simulink model "GCI_Ctrl_PLL_C2000"  (R2024a)
settings: Solver=FixedStepDiscrete  StartTime=0.0  StopTime=8  FixedStep=Sim.ContSampleTime  RelTol=1e-3  EnableMultiTasking=on
values from neighbouring files (symbols this model uses):
  ADPTV = 1.3912    [ModelDD.sldd]
  Ctrl = 0    [ModelDD.sldd]
  EnableMonitors = 0    [ModelDD.sldd]
  FrcPwr = 1    [ModelDD.sldd]
  IdSp = 0.0    [ModelDD.sldd]
  IqSp = 0.0    [ModelDD.sldd]
  ModReq = 1    [ModelDD.sldd]
  PorISel = 0    [ModelDD.sldd]
  PSp = 0.0    [ModelDD.sldd]
  QSp = 0.0    [ModelDD.sldd]
  Sim : value not decoded    [ModelDD.sldd]
  Test = 0    [ModelDD.sldd]
  Var = 650.0    [ModelDD.sldd]
undefined symbols (not defined in the file or in its folder): DiscIntNeverNeededParam, Down, GPTRIP1SEL, GPTRIP2SEL, magnitude, P, TZ1, TZ2, Up
libraries: simulink x38, c2837xDlib x22, c2802xlib x15, slpidlib x9, spsMeanLib x9, spsCurrentMeasurementLib x7, spsThreePhaseVIMeasurementLib x5, spsVoltageMeasurementLib x5, spsTHDLib x4, spsSeriesRLCBranchLib x4, svdutilitieslib x3, c280xlib x3
(part 8 of 11)

== system GCI_Ctrl_PLL_C2000/C2000_SW/CtrlLoop/CurrentController/CurrentControllerAdptv2/MESO/Mag1 ==
  in : Inport
  Gain : Gain  Gain=4
  Gain1 : Gain  Gain=0.5
  Product : Product
  Product1 : Product
  Selector : Selector  NumberOfDimensions=2  InputPortWidth=3  IndexOptions=Index vector (dialog),Index vector (dialog)  Indices=1,1  OutputSizes=1,1
  Selector1 : Selector  NumberOfDimensions=2  InputPortWidth=3  IndexOptions=Index vector (dialog),Index vector (dialog)  Indices=2,2  OutputSizes=1,1
  Selector2 : Selector  NumberOfDimensions=2  InputPortWidth=3  IndexOptions=Index vector (dialog),Index vector (dialog)  Indices=1,2  OutputSizes=1,1
  Selector3 : Selector  NumberOfDimensions=2  InputPortWidth=3  IndexOptions=Index vector (dialog),Index vector (dialog)  Indices=2,1  OutputSizes=1,1
  Sqrt1 : Sqrt
  Sqrt2 : Sqrt
  Square : Math  Operator=square
  Square1 : Math  Operator=square
  Square2 : Math  Operator=square
  Sum : Sum  Inputs=|+-
  Sum of Elements : Sum  Inputs=+
  Sum1 : Sum  Inputs=|+-
  Sum2 : Sum  Inputs=|+-
  Abs : Outport
  wires:
  Sqrt2/1 -> Abs/1
  Gain1/1 -> Sqrt2/1
  Sum2/1 -> Gain1/1
  Sqrt1/1 -> Sum2/2
  Sum1/1 -> Sqrt1/1
  Gain/1 -> Sum1/2
  Square1/1 -> Sum1/1
  Square2/1 -> Gain/1
  [det] -> Square2/1
  Sum/1 -> [det]
  Product1/1 -> Sum/2
  Product/1 -> Sum/1
  Selector2/1 -> Product1/1
  Selector3/1 -> Product1/2
  Selector1/1 -> Product/2
  Selector/1 -> Product/1
  Sum of Elements/1 -> Square1/1, Sum2/1
  in/1 -> Square/1, Selector/1, Selector3/1, Selector2/1, Selector1/1
  Square/1 -> Sum of Elements/1

== system GCI_Ctrl_PLL_C2000/C2000_SW/CtrlLoop/CurrentController/CurrentControllerAdptv2/MESO/Mag2 ==
  in : Inport
  Constant : Constant  OutDataTypeStr=single
  Fcn : Fcn  Expr=(u[2]+sqrt(u[2]^2 - 4*u[1]*u[3]))/(2*u[1])
  Fcn1 : Fcn  Expr=(u[2]-sqrt(u[2]^2 - 4*u[1]*u[3]))/(2*u[1])
  Matrix Multiply : Product  Multiplication=Matrix(*)
  Max : MinMax  Function=max  Inputs=2
  Mux : Mux  Inputs=3
  Product : Product
  Product1 : Product
  Reshape{,1..4} (5 alike) : Reshape
  Selector : Selector  NumberOfDimensions=2  InputPortWidth=3  IndexOptions=Index vector (dialog),Index vector (dialog)  Indices=1,1  OutputSizes=1,1
  Selector1 : Selector  NumberOfDimensions=2  InputPortWidth=3  IndexOptions=Index vector (dialog),Index vector (dialog)  Indices=1,2  OutputSizes=1,1
  Selector2 : Selector  NumberOfDimensions=2  InputPortWidth=3  IndexOptions=Index vector (dialog),Index vector (dialog)  Indices=2,1  OutputSizes=1,1
  Selector3 : Selector  NumberOfDimensions=2  InputPortWidth=3  IndexOptions=Index vector (dialog),Index vector (dialog)  Indices=2,2  OutputSizes=1,1
  Sqrt3 : Sqrt
  Sum : Sum  Inputs=|++
  Sum1 : Sum  Inputs=|+-
  Transpose : matrix_library/Transpose
  Abs : Outport
  wires:
  Matrix Multiply/1 -> Selector/1, Selector1/1, Selector2/1, Selector3/1
  Constant/1 -> Mux/1
  Sum1/1 -> Mux/3
  Product1/1 -> Sum1/2
  Product/1 -> Sum1/1
  Sum/1 -> Mux/2
  Fcn1/1 -> Max/2
  Fcn/1 -> Max/1
  Mux/1 -> Fcn/1, Fcn1/1
  Reshape4/1 -> Sum/2, Product1/2  "d"
  Reshape3/1 -> Product/2  "c"
  Reshape2/1 -> Product/1  "b"
  Selector1/1 -> Reshape2/1
  Selector2/1 -> Reshape3/1
  Selector3/1 -> Reshape4/1
  Reshape1/1 -> Sum/1, Product1/1  "a"
  Selector/1 -> Reshape1/1
  Sqrt3/1 -> Reshape/1
  Max/1 -> Sqrt3/1
  in/1 -> Transpose/1, Matrix Multiply/2
  Transpose/1 -> Matrix Multiply/1
  Reshape/1 -> Abs/1

== system GCI_Ctrl_PLL_C2000/C2000_SW/CtrlLoop/CurrentController/CurrentControllerAdptv2/MESO/Subsystem ==
  $v_k$ : Inport
  "$u_{k-1}$" : Inport  Port=2
  Abs : Abs  SaturateOnIntegerOverflow=off
  Constant : Constant  Value=ADPTV.b_D_ui
  Constant1 : Constant  Value=ADPTV.b_D_ui
  Less Than : RelationalOperator  Operator=<  OutDataTypeStr=boolean  RndMeth=Simplest  InputSameDT=off
  Product : Product
  Sign : Signum
  Sum6 : Sum  Inputs=|++
  Switch : Switch  Criteria=u2 > Threshold  SaturateOnIntegerOverflow=off  InputSameDT=off
  $u_k$ : Outport
  wires:
  "$u_{k-1}$"/1 -> Sum6/2
  Sum6/1 -> $u_k$/1  "$u_k$"
  Switch/1 -> Sum6/1
  Abs/1 -> Less Than/1
  Constant1/1 -> Product/2
  Product/1 -> Switch/3
  Constant/1 -> Less Than/2
  $v_k$/1 -> Switch/1, Abs/1, Sign/1
  Less Than/1 -> [ui_cond]  "$u_{sat}$"
  [ui_cond] -> Switch/2
  Sign/1 -> Product/1

== system GCI_Ctrl_PLL_C2000/C2000_SW/CtrlLoop/CurrentController/CurrentControllerAdptv2/Subsystem/PowerCalculation ==
  VdqP : Inport
  VdqN : Inport  Port=2
  IdqzP : Inport  Port=3
  IdqzN : Inport  Port=4
  Add : Sum  Inputs=-+
  Add3 : Sum
  Add4 : Sum
  Demux : Demux  Outputs=2
  Gain4 : Gain  Gain=1.5  ParamDataTypeStr=single
  Gain5 : Gain  Gain=1.5  ParamDataTypeStr=single
  Product{4..7} (4 alike) : Product
  Selector2 : Selector  InputPortWidth=2  IndexOptions=Index vector (dialog)  Indices=[2 1]  OutputSizes=1
  Selector3 : Selector  InputPortWidth=2  IndexOptions=Index vector (dialog)  Indices=[2 1]  OutputSizes=1
  Sum of Elements3 : Sum  Inputs=+
  P0 : Outport  VectorParamsAs1DForOutWhenUnconnected=off
  Q0 : Outport  Port=2  VectorParamsAs1DForOutWhenUnconnected=off
  wires:
  IdqzP/1 -> [IdqP], Selector2/1
  VdqN/1 -> [VdqN]
  IdqzN/1 -> [IdqN], Selector3/1
  VdqP/1 -> [VdqP]
  Product5/1 -> Add3/2
  Add3/1 -> Demux/1
  Product4/1 -> Add3/1
  Add/1 -> Gain4/1
  Gain4/1 -> Q0/1
  Selector2/1 -> [IqdP]
  Selector3/1 -> [IqdN]
  [IqdP] -> Product4/2
  [VdqP] -> Product4/1
  [IqdN] -> Product5/2
  [VdqN] -> Product5/1
  [VdqN] -> Product7/1
  [IdqN] -> Product7/2
  [VdqP] -> Product6/1
  [IdqP] -> Product6/2
  Gain5/1 -> P0/1
  Sum of Elements3/1 -> Gain5/1
  Product6/1 -> Add4/1
  Add4/1 -> Sum of Elements3/1
  Product7/1 -> Add4/2
  Demux/1 -> Add/1
  Demux/2 -> Add/2

== system GCI_Ctrl_PLL_C2000/C2000_SW/CtrlLoop/CurrentController/CurrentControllerAdptv2/Subsystem/abc_dqz ==
  abc : Inport
  wtNow : Inport  Port=2
  Subsystem : Subsystem
  Subsystem2 : Subsystem
  dqz : Outport  VectorParamsAs1DForOutWhenUnconnected=off
  wires:
  wtNow/1 -> Subsystem2/2(Ang)
  abc/1 -> Subsystem/1(abc)
  Subsystem/1(al_be_0) -> Subsystem2/1(alpha_beta)
  Subsystem2/1(dq) -> dqz/1

== system GCI_Ctrl_PLL_C2000/C2000_SW/CtrlLoop/CurrentController/CurrentControllerAdptv2/Subsystem/abc_dqz1 ==
  abc : Inport
  wtNow : Inport  Port=2
  Subsystem : Subsystem
  Subsystem2 : Subsystem
  dqz : Outport  VectorParamsAs1DForOutWhenUnconnected=off
  wires:
  Subsystem2/1(dq) -> dqz/1
  Subsystem/1(al_be_0) -> Subsystem2/1(alpha_beta)
  abc/1 -> Subsystem/1(abc)
  wtNow/1 -> Subsystem2/2(Ang)

== system GCI_Ctrl_PLL_C2000/C2000_SW/CtrlLoop/CurrentController/CurrentControllerAdptv2/Subsystem/dd_dqz1 ==
  abc : Inport
  wtNow : Inport  Port=2
  Delay : Delay  DelayLength=1
  Delay1 : Delay  DelayLength=1
  Gain : Gain  Gain=-1  ParamDataTypeStr=single
  LPF : Subsystem  mask{Ts=1/(Var.PWM_Freq), w=single(2*pi*50), K=single(1), y_0=0}
      mask prompts: Ts "Sample Time (s)"; w "CutOff Freq (-3db) (rad/s)"; K "Gain"; y_0 "Initial output"
  LPF1 : Subsystem  mask{Ts=1/(Var.PWM_Freq), w=single(2*pi*50), K=single(1), y_0=0}
      mask prompts: Ts "Sample Time (s)"; w "CutOff Freq (-3db) (rad/s)"; K "Gain"; y_0 "Initial output"
  Subsystem : Subsystem
  Subsystem1 : Subsystem
  Subsystem2 : Subsystem
  Subsystem3 : Subsystem
  Subsystem4 : Subsystem
  dqzP : Outport  VectorParamsAs1DForOutWhenUnconnected=off
  dqzN : Outport  Port=2  VectorParamsAs1DForOutWhenUnconnected=off
  wires:
  Subsystem1/1(dq) -> Subsystem3/1(Vdq_in)
  Subsystem2/1(dq) -> Subsystem4/1(Vdq_in)
  Subsystem4/1(Vdq_out) -> LPF/1(u), dqzP/1
  Delay/1 -> Subsystem3/2(Vdq_Inverse)
  Delay1/1 -> Subsystem4/2(Vdq_Inverse)
  Subsystem3/1(Vdq_out) -> LPF1/1(u), dqzN/1
  LPF1/1(y) -> Delay1/1
  LPF/1(y) -> Delay/1
  Gain/1 -> Subsystem1/2(wtNow), Subsystem3/3(Theta)
  abc/1 -> Subsystem/1(abc)
  Subsystem/1(al_be_0) -> Subsystem2/1(alpha_beta), Subsystem1/1(alpha_beta)
  wtNow/1 -> Gain/1, Subsystem2/2(wtNow), Subsystem4/3(Theta)

== system GCI_Ctrl_PLL_C2000/C2000_SW/CtrlLoop/CurrentController/CurrentControllerAdptv2/Subsystem/dd_dqz2 ==
  abc : Inport
  wtNow : Inport  Port=2
  Delay : Delay  DelayLength=1
  Delay1 : Delay  DelayLength=1
  Gain : Gain  Gain=-1  ParamDataTypeStr=single
  LPF : Subsystem  mask{Ts=1/(Var.PWM_Freq), w=single(50), K=single(1), y_0=0}
      mask prompts: Ts "Sample Time (s)"; w "CutOff Freq (-3db) (rad/s)"; K "Gain"; y_0 "Initial output"
  LPF1 : Subsystem  mask{Ts=1/(Var.PWM_Freq), w=single(50), K=single(1), y_0=0}
      mask prompts: Ts "Sample Time (s)"; w "CutOff Freq (-3db) (rad/s)"; K "Gain"; y_0 "Initial output"
  Subsystem : Subsystem
  Subsystem1 : Subsystem
  Subsystem2 : Subsystem
  Subsystem3 : Subsystem
  Subsystem4 : Subsystem
  dqzP : Outport  VectorParamsAs1DForOutWhenUnconnected=off
  dqzN : Outport  Port=2  VectorParamsAs1DForOutWhenUnconnected=off
  wires:
  Subsystem/1(al_be_0) -> Subsystem1/1(alpha_beta), Subsystem2/1(alpha_beta)
  abc/1 -> Subsystem/1(abc)
  Gain/1 -> Subsystem3/3(Theta), Subsystem1/2(wtNow)
  LPF/1(y) -> Delay/1
  LPF1/1(y) -> Delay1/1
  Subsystem3/1(Vdq_out) -> LPF1/1(u), dqzN/1
  Delay1/1 -> Subsystem4/2(Vdq_Inverse)
  Delay/1 -> Subsystem3/2(Vdq_Inverse)
  Subsystem4/1(Vdq_out) -> LPF/1(u), dqzP/1
  Subsystem2/1(dq) -> Subsystem4/1(Vdq_in)
  Subsystem1/1(dq) -> Subsystem3/1(Vdq_in)
  wtNow/1 -> Gain/1, Subsystem4/3(Theta), Subsystem2/2(wtNow)

== system GCI_Ctrl_PLL_C2000/C2000_SW/CtrlLoop/CurrentController/CurrentControllerAdptv2/dqz2abc_1/Subsystem ==
  al_be_0 : Inport  OutDataTypeStr=single  PortDimensions=3
  Gain3 : Gain  Gain="single([ 1   0   1; -1/2  sqrt(3)/2   1; -1/2  -sqrt(3)/2  1 ] )"  Multiplication=Matrix(K*u) (u vector)  ParamDataTypeStr=single  OutDataTypeStr=single  SaturateOnIntegerOverflow=on
  abc : Outport  OutDataTypeStr=single  VectorParamsAs1DForOutWhenUnconnected=off
  wires:
  al_be_0/1 -> Gain3/1
  Gain3/1 -> abc/1  "abc"

== system GCI_Ctrl_PLL_C2000/C2000_SW/CtrlLoop/CurrentController/CurrentControllerAdptv2/dqz2abc_1/Subsystem1 ==
  note: =
  note: =
  note: *
  note: [ d
      |    q ]
  note: [  al
      |     be  ]
  note: [ d
      |    q ]
  note: inv ([  cos(wt)   sin(wt)
      |    -sin(wt)    cos(wt)   ])
  note: [  al
      |     be  ]
  note: [  cos(wt)   -sin(wt)
      |    sin(wt)    cos(wt)   ]
  note: *
  dqz : Inport  OutDataTypeStr=single  PortDimensions=3
  Ang : Inport  Port=2  OutDataTypeStr=single  PortDimensions=1
  Fcn : Fcn  Expr=u[1]*cos(u[3]) - u[2]*sin(u[3])
  Fcn1 : Fcn  Expr=u[1]*sin(u[3]) + u[2]*cos(u[3])
  Mux1 : Mux  Inputs=3
  Mux2 : Mux  Inputs=[2 1]
  Mux3 : Mux  Inputs=[2 1]
  Selector : Selector  InputPortWidth=3  IndexOptions=Index vector (dialog)  Indices=[1 2]  OutputSizes=1
  Selector1 : Selector  InputPortWidth=3  IndexOptions=Index vector (dialog)  Indices=[3]  OutputSizes=1
  alpha_beta : Outport  OutDataTypeStr=single  InitialOutput=[0,0]  VectorParamsAs1DForOutWhenUnconnected=off
  wires:
  Selector1/1 -> Mux1/3
  dqz/1 -> Selector/1, Selector1/1
  Selector/1 -> Mux3/1, Mux2/1
  Fcn/1 -> Mux1/1
  Ang/1 -> Mux3/2, Mux2/2
  Mux2/1 -> Fcn/1
  Mux1/1 -> alpha_beta/1
  Mux3/1 -> Fcn1/1
  Fcn1/1 -> Mux1/2

== system GCI_Ctrl_PLL_C2000/C2000_SW/CtrlLoop/CurrentController/CurrentControllerPosNegSeq/Phase2Line/Line ==
  In : Inport
  Demux : Demux  Outputs=3
  Gain : Gain  Gain=single(1/3)  ParamDataTypeStr=single
  Gain1 : Gain  Gain=single(1/3)  ParamDataTypeStr=single
  Gain2 : Gain  Gain=single(1/3)  ParamDataTypeStr=single
  Mux : Mux  Inputs=3
  Sum : Sum  Inputs=|+-
  Sum1 : Sum  Inputs=-+|
  Sum2 : Sum  Inputs=-+|
  Out : Outport
  wires:
  In/1 -> Demux/1
  Demux/1 -> Sum1/1, Sum/1
  Demux/3 -> Sum2/2, Sum/2
  Demux/2 -> Sum2/1, Sum1/2
  Sum/1 -> Gain/1
  Sum2/1 -> Gain2/1
  Sum1/1 -> Gain1/1
  Gain1/1 -> Mux/2
  Gain2/1 -> Mux/3
  Gain/1 -> Mux/1
  Mux/1 -> Out/1

== system GCI_Ctrl_PLL_C2000/C2000_SW/CtrlLoop/CurrentController/CurrentControllerPosNegSeq/Phase2Line/Phase ==
  In : Inport
  Out : Outport
  wires:
  In/1 -> Out/1

== system GCI_Ctrl_PLL_C2000/C2000_SW/CtrlLoop/CurrentController/CurrentControllerPosNegSeq/Subsystem/PowerCalculation ==
  VdqP : Inport
  VdqN : Inport  Port=2
  IdqzP : Inport  Port=3
  IdqzN : Inport  Port=4
  Add : Sum  Inputs=-+
  Add3 : Sum
  Add4 : Sum
  Demux : Demux  Outputs=2
  Gain4 : Gain  Gain=1.5  ParamDataTypeStr=single
  Gain5 : Gain  Gain=1.5  ParamDataTypeStr=single
  Product{4..7} (4 alike) : Product
  Selector2 : Selector  InputPortWidth=2  IndexOptions=Index vector (dialog)  Indices=[2 1]  OutputSizes=1
  Selector3 : Selector  InputPortWidth=2  IndexOptions=Index vector (dialog)  Indices=[2 1]  OutputSizes=1
  Sum of Elements3 : Sum  Inputs=+
  P0 : Outport  VectorParamsAs1DForOutWhenUnconnected=off
  Q0 : Outport  Port=2  VectorParamsAs1DForOutWhenUnconnected=off
  wires:
  IdqzP/1 -> [IdqP], Selector2/1
  VdqN/1 -> [VdqN]
  IdqzN/1 -> [IdqN], Selector3/1
  VdqP/1 -> [VdqP]
  Product5/1 -> Add3/2
  Add3/1 -> Demux/1
  Product4/1 -> Add3/1
  Add/1 -> Gain4/1
  Gain4/1 -> Q0/1
  Selector2/1 -> [IqdP]
  Selector3/1 -> [IqdN]
  [IqdP] -> Product4/2
  [VdqP] -> Product4/1
  [IqdN] -> Product5/2
  [VdqN] -> Product5/1
  [VdqN] -> Product7/1
  [IdqN] -> Product7/2
  [VdqP] -> Product6/1
  [IdqP] -> Product6/2
  Gain5/1 -> P0/1
  Sum of Elements3/1 -> Gain5/1
  Product6/1 -> Add4/1
  Add4/1 -> Sum of Elements3/1
  Product7/1 -> Add4/2
  Demux/1 -> Add/1
  Demux/2 -> Add/2

== system GCI_Ctrl_PLL_C2000/C2000_SW/CtrlLoop/CurrentController/CurrentControllerPosNegSeq/Subsystem/abc_dqz ==
  abc : Inport
  wtNow : Inport  Port=2
  Subsystem : Subsystem
  Subsystem2 : Subsystem
  dqz : Outport  VectorParamsAs1DForOutWhenUnconnected=off
  wires:
  wtNow/1 -> Subsystem2/2(Ang)
  abc/1 -> Subsystem/1(abc)
  Subsystem/1(al_be_0) -> Subsystem2/1(alpha_beta)
  Subsystem2/1(dq) -> dqz/1

== system GCI_Ctrl_PLL_C2000/C2000_SW/CtrlLoop/CurrentController/CurrentControllerPosNegSeq/Subsystem/dd_dqz1 ==
  abc : Inport
  wtNow : Inport  Port=2
  Delay : Delay  DelayLength=1
  Delay1 : Delay  DelayLength=1
  Gain : Gain  Gain=-1  ParamDataTypeStr=single
  LPF : Subsystem  mask{Ts=1/(Var.PWM_Freq), w=single(2*pi*50), K=single(1), y_0=0}
      mask prompts: Ts "Sample Time (s)"; w "CutOff Freq (-3db) (rad/s)"; K "Gain"; y_0 "Initial output"
  LPF1 : Subsystem  mask{Ts=1/(Var.PWM_Freq), w=single(2*pi*50), K=single(1), y_0=0}
      mask prompts: Ts "Sample Time (s)"; w "CutOff Freq (-3db) (rad/s)"; K "Gain"; y_0 "Initial output"
  Subsystem : Subsystem
  Subsystem1 : Subsystem
  Subsystem2 : Subsystem
  Subsystem3 : Subsystem
  Subsystem4 : Subsystem
  dqzP : Outport  VectorParamsAs1DForOutWhenUnconnected=off
  dqzN : Outport  Port=2  VectorParamsAs1DForOutWhenUnconnected=off
  wires:
  Subsystem1/1(dq) -> Subsystem3/1(Vdq_in)
  Subsystem2/1(dq) -> Subsystem4/1(Vdq_in)
  Subsystem4/1(Vdq_out) -> LPF/1(u), dqzP/1
  Delay/1 -> Subsystem3/2(Vdq_Inverse)
  Delay1/1 -> Subsystem4/2(Vdq_Inverse)
  Subsystem3/1(Vdq_out) -> LPF1/1(u), dqzN/1
  LPF1/1(y) -> Delay1/1
  LPF/1(y) -> Delay/1
  Gain/1 -> Subsystem1/2(wtNow), Subsystem3/3(Theta)
  abc/1 -> Subsystem/1(abc)
  Subsystem/1(al_be_0) -> Subsystem2/1(alpha_beta), Subsystem1/1(alpha_beta)
  wtNow/1 -> Gain/1, Subsystem2/2(wtNow), Subsystem4/3(Theta)

== system GCI_Ctrl_PLL_C2000/C2000_SW/CtrlLoop/CurrentController/CurrentControllerPosNegSeq/Subsystem/dd_dqz2 ==
  abc : Inport
  wtNow : Inport  Port=2
  Delay : Delay  DelayLength=1
  Delay1 : Delay  DelayLength=1
  Gain : Gain  Gain=-1  ParamDataTypeStr=single
  LPF : Subsystem  mask{Ts=1/(Var.PWM_Freq), w=single(50), K=single(1), y_0=0}
      mask prompts: Ts "Sample Time (s)"; w "CutOff Freq (-3db) (rad/s)"; K "Gain"; y_0 "Initial output"
  LPF1 : Subsystem  mask{Ts=1/(Var.PWM_Freq), w=single(50), K=single(1), y_0=0}
      mask prompts: Ts "Sample Time (s)"; w "CutOff Freq (-3db) (rad/s)"; K "Gain"; y_0 "Initial output"
  Subsystem : Subsystem
  Subsystem1 : Subsystem
  Subsystem2 : Subsystem
  Subsystem3 : Subsystem
  Subsystem4 : Subsystem
  dqzP : Outport  VectorParamsAs1DForOutWhenUnconnected=off
  dqzN : Outport  Port=2  VectorParamsAs1DForOutWhenUnconnected=off
  wires:
  Subsystem/1(al_be_0) -> Subsystem1/1(alpha_beta), Subsystem2/1(alpha_beta)
  abc/1 -> Subsystem/1(abc)
  Gain/1 -> Subsystem3/3(Theta), Subsystem1/2(wtNow)
  LPF/1(y) -> Delay/1
  LPF1/1(y) -> Delay1/1
  Subsystem3/1(Vdq_out) -> LPF1/1(u), dqzN/1
  Delay1/1 -> Subsystem4/2(Vdq_Inverse)
  Delay/1 -> Subsystem3/2(Vdq_Inverse)
  Subsystem4/1(Vdq_out) -> LPF/1(u), dqzP/1
  Subsystem2/1(dq) -> Subsystem4/1(Vdq_in)
  Subsystem1/1(dq) -> Subsystem3/1(Vdq_in)
  wtNow/1 -> Gain/1, Subsystem4/3(Theta), Subsystem2/2(wtNow)

== system GCI_Ctrl_PLL_C2000/C2000_SW/CtrlLoop/CurrentController/CurrentControllerPosNegSeq/dqz2abc_1/Subsystem ==
  al_be_0 : Inport  OutDataTypeStr=single  PortDimensions=3
  Gain3 : Gain  Gain="single([ 1   0   1; -1/2  sqrt(3)/2   1; -1/2  -sqrt(3)/2  1 ] )"  Multiplication=Matrix(K*u) (u vector)  ParamDataTypeStr=single  OutDataTypeStr=single  SaturateOnIntegerOverflow=on
  abc : Outport  OutDataTypeStr=single  VectorParamsAs1DForOutWhenUnconnected=off
  wires:
  al_be_0/1 -> Gain3/1
  Gain3/1 -> abc/1  "abc"

== system GCI_Ctrl_PLL_C2000/C2000_SW/CtrlLoop/CurrentController/CurrentControllerPosNegSeq/dqz2abc_1/Subsystem1 ==
  note: =
  note: =
  note: *
  note: [ d
      |    q ]
  note: [  al
      |     be  ]
  note: [ d
      |    q ]
  note: inv ([  cos(wt)   sin(wt)
      |    -sin(wt)    cos(wt)   ])
  note: [  al
      |     be  ]
  note: [  cos(wt)   -sin(wt)
      |    sin(wt)    cos(wt)   ]
  note: *
  dqz : Inport  OutDataTypeStr=single  PortDimensions=3
  Ang : Inport  Port=2  OutDataTypeStr=single  PortDimensions=1
  Fcn : Fcn  Expr=u[1]*cos(u[3]) - u[2]*sin(u[3])
  Fcn1 : Fcn  Expr=u[1]*sin(u[3]) + u[2]*cos(u[3])
  Mux1 : Mux  Inputs=3
  Mux2 : Mux  Inputs=[2 1]
  Mux3 : Mux  Inputs=[2 1]
  Selector : Selector  InputPortWidth=3  IndexOptions=Index vector (dialog)  Indices=[1 2]  OutputSizes=1
  Selector1 : Selector  InputPortWidth=3  IndexOptions=Index vector (dialog)  Indices=[3]  OutputSizes=1
  alpha_beta : Outport  OutDataTypeStr=single  InitialOutput=[0,0]  VectorParamsAs1DForOutWhenUnconnected=off
  wires:
  Selector1/1 -> Mux1/3
  dqz/1 -> Selector/1, Selector1/1
  Selector/1 -> Mux3/1, Mux2/1
  Fcn/1 -> Mux1/1
  Ang/1 -> Mux3/2, Mux2/2
  Mux2/1 -> Fcn/1
  Mux1/1 -> alpha_beta/1
  Mux3/1 -> Fcn1/1
  Fcn1/1 -> Mux1/2

== system GCI_Ctrl_PLL_C2000/C2000_SW/CtrlLoop/CurrentController/CurrentControllerPosNegSeq/dqz2abc_2/Subsystem ==
  al_be_0 : Inport  OutDataTypeStr=single  PortDimensions=3
  Gain3 : Gain  Gain="single([ 1   0   1; -1/2  sqrt(3)/2   1; -1/2  -sqrt(3)/2  1 ] )"  Multiplication=Matrix(K*u) (u vector)  ParamDataTypeStr=single  OutDataTypeStr=single  SaturateOnIntegerOverflow=on
  abc : Outport  OutDataTypeStr=single  VectorParamsAs1DForOutWhenUnconnected=off
  wires:
  Gain3/1 -> abc/1
  al_be_0/1 -> Gain3/1

== system GCI_Ctrl_PLL_C2000/C2000_SW/CtrlLoop/CurrentController/CurrentControllerPosNegSeq/dqz2abc_2/Subsystem1 ==
  note: *
  note: [  cos(wt)   -sin(wt)
      |    sin(wt)    cos(wt)   ]
  note: [  al
      |     be  ]
  note: inv ([  cos(wt)   sin(wt)
      |    -sin(wt)    cos(wt)   ])
  note: [ d
      |    q ]
  note: [  al
      |     be  ]
  note: [ d
      |    q ]
  note: *
  note: =
  note: =
  dqz : Inport  OutDataTypeStr=single  PortDimensions=3
  Ang : Inport  Port=2  OutDataTypeStr=single  PortDimensions=1
  Fcn : Fcn  Expr=u[1]*cos(u[3]) - u[2]*sin(u[3])
  Fcn1 : Fcn  Expr=u[1]*sin(u[3]) + u[2]*cos(u[3])
  Mux1 : Mux  Inputs=3
  Mux2 : Mux  Inputs=[2 1]
  Mux3 : Mux  Inputs=[2 1]
  Selector : Selector  InputPortWidth=3  IndexOptions=Index vector (dialog)  Indices=[1 2]  OutputSizes=1
  Selector1 : Selector  InputPortWidth=3  IndexOptions=Index vector (dialog)  Indices=[3]  OutputSizes=1
  alpha_beta : Outport  OutDataTypeStr=single  InitialOutput=[0,0]  VectorParamsAs1DForOutWhenUnconnected=off
  wires:
  Fcn1/1 -> Mux1/2
  Mux3/1 -> Fcn1/1
  Mux1/1 -> alpha_beta/1
  Mux2/1 -> Fcn/1
  Ang/1 -> Mux2/2, Mux3/2
  Fcn/1 -> Mux1/1
  Selector/1 -> Mux2/1, Mux3/1
  dqz/1 -> Selector1/1, Selector/1
  Selector1/1 -> Mux1/3

== system GCI_Ctrl_PLL_C2000/C2000_SW/CtrlLoop/CurrentController/FeedForward/Subsystem/LPF ==
  u : Inport
  Alpha : Gain  Gain=(2-w*Ts)/(2+w*Ts)
  Beta : Gain  Gain=(w*Ts)/(2+w*Ts)
  Delay1 : Delay  DelayLength=1  InitialCondition=y_0
  Delay2 : Delay  DelayLength=1
  Sum1 : Sum  Inputs=++|
  Sum2 : Sum  Inputs=|++
  y : Outport  VectorParamsAs1DForOutWhenUnconnected=off
  wires:
  u/1 -> Sum1/1, Delay2/1
  Delay1/1 -> Alpha/1  "y(n-1)"
  Alpha/1 -> Sum2/2
  Delay2/1 -> Sum1/2
  Sum1/1 -> Beta/1
  Beta/1 -> Sum2/1
  Sum2/1 -> Delay1/1, y/1

== system GCI_Ctrl_PLL_C2000/C2000_SW/CtrlLoop/CurrentController/FeedForward/Subsystem/LPF1 ==
  u : Inport
  Alpha : Gain  Gain=(2-w*Ts)/(2+w*Ts)
  Beta : Gain  Gain=(w*Ts)/(2+w*Ts)
  Delay1 : Delay  DelayLength=1  InitialCondition=y_0
  Delay2 : Delay  DelayLength=1
  Sum1 : Sum  Inputs=++|
  Sum2 : Sum  Inputs=|++
  y : Outport  VectorParamsAs1DForOutWhenUnconnected=off
  wires:
  Sum2/1 -> y/1, Delay1/1
  Beta/1 -> Sum2/1
  Sum1/1 -> Beta/1
  Delay2/1 -> Sum1/2
  Alpha/1 -> Sum2/2
  Delay1/1 -> Alpha/1  "y(n-1)"
  u/1 -> Delay2/1, Sum1/1

== system GCI_Ctrl_PLL_C2000/C2000_SW/CtrlLoop/CurrentController/FeedForward/Subsystem/PowerCalculation ==
  VdqP : Inport
  VdqN : Inport  Port=2
  IdqzP : Inport  Port=3
  IdqzN : Inport  Port=4
  Add : Sum  Inputs=-+
  Add3 : Sum
  Add4 : Sum
  Demux : Demux  Outputs=2
  Gain4 : Gain  Gain=1.5  ParamDataTypeStr=single
  Gain5 : Gain  Gain=1.5  ParamDataTypeStr=single
  Product{4..7} (4 alike) : Product
  Selector2 : Selector  InputPortWidth=2  IndexOptions=Index vector (dialog)  Indices=[2 1]  OutputSizes=1
  Selector3 : Selector  InputPortWidth=2  IndexOptions=Index vector (dialog)  Indices=[2 1]  OutputSizes=1
  Sum of Elements3 : Sum  Inputs=+
  P0 : Outport  VectorParamsAs1DForOutWhenUnconnected=off
  Q0 : Outport  Port=2  VectorParamsAs1DForOutWhenUnconnected=off
  wires:
  IdqzP/1 -> [IdqP], Selector2/1
  VdqN/1 -> [VdqN]
  IdqzN/1 -> [IdqN], Selector3/1
  VdqP/1 -> [VdqP]
  Product5/1 -> Add3/2
  Add3/1 -> Demux/1
  Product4/1 -> Add3/1
  Add/1 -> Gain4/1
  Gain4/1 -> Q0/1
  Selector2/1 -> [IqdP]
  Selector3/1 -> [IqdN]
  [IqdP] -> Product4/2
  [VdqP] -> Product4/1
  [IqdN] -> Product5/2
  [VdqN] -> Product5/1
  [VdqN] -> Product7/1
  [IdqN] -> Product7/2
  [VdqP] -> Product6/1
  [IdqP] -> Product6/2
  Gain5/1 -> P0/1
  Sum of Elements3/1 -> Gain5/1
  Product6/1 -> Add4/1
  Add4/1 -> Sum of Elements3/1
  Product7/1 -> Add4/2
  Demux/1 -> Add/1
  Demux/2 -> Add/2

== system GCI_Ctrl_PLL_C2000/C2000_SW/CtrlLoop/CurrentController/FeedForward/Subsystem/abc_dqz ==
  abc : Inport
  wtNow : Inport  Port=2
  Subsystem : Subsystem
  Subsystem2 : Subsystem
  dqz : Outport  VectorParamsAs1DForOutWhenUnconnected=off
  wires:
  wtNow/1 -> Subsystem2/2(Ang)
  abc/1 -> Subsystem/1(abc)
  Subsystem/1(al_be_0) -> Subsystem2/1(alpha_beta)
  Subsystem2/1(dq) -> dqz/1

== system GCI_Ctrl_PLL_C2000/C2000_SW/CtrlLoop/CurrentController/FeedForward/Subsystem/dd_dqz1 ==
  abc : Inport
  wtNow : Inport  Port=2
  Delay : Delay  DelayLength=1
  Delay1 : Delay  DelayLength=1
  Gain : Gain  Gain=-1  ParamDataTypeStr=single
  LPF : Subsystem  mask{Ts=1/(Var.PWM_Freq), w=single(2*pi*50), K=single(1), y_0=0}
      mask prompts: Ts "Sample Time (s)"; w "CutOff Freq (-3db) (rad/s)"; K "Gain"; y_0 "Initial output"
  LPF1 : Subsystem  mask{Ts=1/(Var.PWM_Freq), w=single(2*pi*50), K=single(1), y_0=0}
      mask prompts: Ts "Sample Time (s)"; w "CutOff Freq (-3db) (rad/s)"; K "Gain"; y_0 "Initial output"
  Subsystem : Subsystem
  Subsystem1 : Subsystem
  Subsystem2 : Subsystem
  Subsystem3 : Subsystem
  Subsystem4 : Subsystem
  dqzP : Outport  VectorParamsAs1DForOutWhenUnconnected=off
  dqzN : Outport  Port=2  VectorParamsAs1DForOutWhenUnconnected=off
  wires:
  Subsystem1/1(dq) -> Subsystem3/1(Vdq_in)
  Subsystem2/1(dq) -> Subsystem4/1(Vdq_in)
  Subsystem4/1(Vdq_out) -> LPF/1(u), dqzP/1
  Delay/1 -> Subsystem3/2(Vdq_Inverse)
  Delay1/1 -> Subsystem4/2(Vdq_Inverse)
  Subsystem3/1(Vdq_out) -> LPF1/1(u), dqzN/1
  LPF1/1(y) -> Delay1/1
  LPF/1(y) -> Delay/1
  Gain/1 -> Subsystem1/2(wtNow), Subsystem3/3(Theta)
  abc/1 -> Subsystem/1(abc)
  Subsystem/1(al_be_0) -> Subsystem2/1(alpha_beta), Subsystem1/1(alpha_beta)
  wtNow/1 -> Gain/1, Subsystem2/2(wtNow), Subsystem4/3(Theta)

== system GCI_Ctrl_PLL_C2000/C2000_SW/CtrlLoop/CurrentController/FeedForward/Subsystem/dd_dqz2 ==
  abc : Inport
  wtNow : Inport  Port=2
  Delay : Delay  DelayLength=1
  Delay1 : Delay  DelayLength=1
  Gain : Gain  Gain=-1  ParamDataTypeStr=single
  LPF : Subsystem  mask{Ts=1/(Var.PWM_Freq), w=single(50), K=single(1), y_0=0}
      mask prompts: Ts "Sample Time (s)"; w "CutOff Freq (-3db) (rad/s)"; K "Gain"; y_0 "Initial output"
  LPF1 : Subsystem  mask{Ts=1/(Var.PWM_Freq), w=single(50), K=single(1), y_0=0}
      mask prompts: Ts "Sample Time (s)"; w "CutOff Freq (-3db) (rad/s)"; K "Gain"; y_0 "Initial output"
  Subsystem : Subsystem
  Subsystem1 : Subsystem
  Subsystem2 : Subsystem
  Subsystem3 : Subsystem
  Subsystem4 : Subsystem
  dqzP : Outport  VectorParamsAs1DForOutWhenUnconnected=off
  dqzN : Outport  Port=2  VectorParamsAs1DForOutWhenUnconnected=off
  wires:
  Subsystem/1(al_be_0) -> Subsystem1/1(alpha_beta), Subsystem2/1(alpha_beta)
  abc/1 -> Subsystem/1(abc)
  Gain/1 -> Subsystem3/3(Theta), Subsystem1/2(wtNow)
  LPF/1(y) -> Delay/1
  LPF1/1(y) -> Delay1/1
  Subsystem3/1(Vdq_out) -> LPF1/1(u), dqzN/1
  Delay1/1 -> Subsystem4/2(Vdq_Inverse)
  Delay/1 -> Subsystem3/2(Vdq_Inverse)
  Subsystem4/1(Vdq_out) -> LPF/1(u), dqzP/1
  Subsystem2/1(dq) -> Subsystem4/1(Vdq_in)
  Subsystem1/1(dq) -> Subsystem3/1(Vdq_in)
  wtNow/1 -> Gain/1, Subsystem4/3(Theta), Subsystem2/2(wtNow)

== system GCI_Ctrl_PLL_C2000/C2000_SW/CtrlLoop/PLL_Vref/SRF_PLL/WrapedDiscIntegrator/WrapZeroToTwoPi ==
  Ang : Inport
  Constant2 : Constant  Value=single(2*pi)  OutDataTypeStr=single
  Mod1 : Math  Operator=mod  SignedPower=on  OutDataTypeStr=single
  wtWraped : Outport  VectorParamsAs1DForOutWhenUnconnected=off
  wires:
  Constant2/1 -> Mod1/2
  Mod1/1 -> wtWraped/1  "Ang"
  Ang/1 -> Mod1/1

== system GCI_Ctrl_PLL_C2000/C2000_SW/CtrlLoop/PLL_Vref/Subsystem/abc_dqz/Subsystem ==
  abc : Inport  PortDimensions=3
  Gain1 : Gain  Gain=single(2/3)  ParamDataTypeStr=single  SaturateOnIntegerOverflow=on  OutDataTypeStr=Inherit: Same as input
  Gain3 : Gain  Gain="single([ 1   -1/2   -1/2; 0   sqrt(3)/2   -sqrt(3)/2; 1/2  1/2  1/2 ] )"  Multiplication=Matrix(K*u) (u vector)  ParamDataTypeStr=single  SaturateOnIntegerOverflow=on  OutDataTypeStr=Inherit: Same as input
  al_be_0 : Outport  VectorParamsAs1DForOutWhenUnconnected=off
  wires:
  abc/1 -> Gain3/1
  Gain3/1 -> Gain1/1
  Gain1/1 -> al_be_0/1

== system GCI_Ctrl_PLL_C2000/C2000_SW/CtrlLoop/PLL_Vref/Subsystem/abc_dqz/Subsystem2 ==
  note: [  al
      |     be  ]
  note: q = -al*sin(wt) + be*cos(wt)
  note: [  cos(wt)   sin(wt)
      |    -sin(wt)    cos(wt)   ]
  note: d = al*cos(wt) + be*sin(wt)
  note: [ d
      |    q ]
  note: *
  note: =
  alpha_beta : Inport
  Ang : Inport  Port=2  PortDimensions=1
  Fcn : Fcn  Expr=u[1]*cos(u[3]) + u[2]*sin(u[3])
  Fcn1 : Fcn  Expr=-u[1]*sin(u[3]) + u[2]*cos(u[3])
  Mux : Mux  Inputs=3
  Mux1 : Mux  Inputs=[2 1]
  Mux2 : Mux  Inputs=[2 1]
  Selector : Selector  InputPortWidth=3  IndexOptions=Index vector (dialog)  Indices=[1 2]  OutputSizes=1
  Selector1 : Selector  InputPortWidth=3  IndexOptions=Index vector (dialog)  Indices=[3]  OutputSizes=1
  dq : Outport  InitialOutput=[0,0]  VectorParamsAs1DForOutWhenUnconnected=off
  wires:
  Selector1/1 -> Mux/3
  Selector/1 -> Mux1/1, Mux2/1
  Mux2/1 -> Fcn1/1
  Mux/1 -> dq/1
  Ang/1 -> Mux1/2, Mux2/2
  Fcn/1 -> Mux/1
  Fcn1/1 -> Mux/2
  Mux1/1 -> Fcn/1
  alpha_beta/1 -> Selector1/1, Selector/1

== system GCI_Ctrl_PLL_C2000/C2000_SW/CtrlLoop/PLL_Vref/Subsystem/dd_dqz1/LPF ==
  u : Inport
  Alpha : Gain  Gain=(2-w*Ts)/(2+w*Ts)
  Beta : Gain  Gain=(w*Ts)/(2+w*Ts)
  Delay1 : Delay  DelayLength=1  InitialCondition=y_0
  Delay2 : Delay  DelayLength=1
  Sum1 : Sum  Inputs=++|
  Sum2 : Sum  Inputs=|++
  y : Outport  VectorParamsAs1DForOutWhenUnconnected=off
  wires:
  u/1 -> Sum1/1, Delay2/1
  Delay1/1 -> Alpha/1  "y(n-1)"
  Alpha/1 -> Sum2/2
  Delay2/1 -> Sum1/2
  Sum1/1 -> Beta/1
  Beta/1 -> Sum2/1
  Sum2/1 -> Delay1/1, y/1

== system GCI_Ctrl_PLL_C2000/C2000_SW/CtrlLoop/PLL_Vref/Subsystem/dd_dqz1/LPF1 ==
  u : Inport
  Alpha : Gain  Gain=(2-w*Ts)/(2+w*Ts)
  Beta : Gain  Gain=(w*Ts)/(2+w*Ts)
  Delay1 : Delay  DelayLength=1  InitialCondition=y_0
  Delay2 : Delay  DelayLength=1
  Sum1 : Sum  Inputs=++|
  Sum2 : Sum  Inputs=|++
  y : Outport  VectorParamsAs1DForOutWhenUnconnected=off
  wires:
  Sum2/1 -> y/1, Delay1/1
  Beta/1 -> Sum2/1
  Sum1/1 -> Beta/1
  Delay2/1 -> Sum1/2
  Alpha/1 -> Sum2/2
  Delay1/1 -> Alpha/1  "y(n-1)"
  u/1 -> Delay2/1, Sum1/1

== system GCI_Ctrl_PLL_C2000/C2000_SW/CtrlLoop/PLL_Vref/Subsystem/dd_dqz1/Subsystem ==
  abc : Inport  PortDimensions=3
  Gain1 : Gain  Gain=single(2/3)  ParamDataTypeStr=single  SaturateOnIntegerOverflow=on  OutDataTypeStr=Inherit: Same as input
  Gain3 : Gain  Gain="single([ 1   -1/2   -1/2; 0   sqrt(3)/2   -sqrt(3)/2; 1/2  1/2  1/2 ] )"  Multiplication=Matrix(K*u) (u vector)  ParamDataTypeStr=single  SaturateOnIntegerOverflow=on  OutDataTypeStr=Inherit: Same as input
  al_be_0 : Outport  VectorParamsAs1DForOutWhenUnconnected=off
  wires:
  abc/1 -> Gain3/1
  Gain3/1 -> Gain1/1
  Gain1/1 -> al_be_0/1  "AlphaBetaZero"

== system GCI_Ctrl_PLL_C2000/C2000_SW/CtrlLoop/PLL_Vref/Subsystem/dd_dqz1/Subsystem1 ==
  note: =
  note: *
  note: [ d
      |    q ]
  note: d = al*cos(wt) + be*sin(wt)
  note: [  cos(wt)   sin(wt)
      |    -sin(wt)    cos(wt)   ]
  note: q = -al*sin(wt) + be*cos(wt)
  note: [  al
      |     be  ]
  alpha_beta : Inport
  wtNow : Inport  Port=2  PortDimensions=1
  Fcn : Fcn  Expr=u[1]*cos(u[3]) + u[2]*sin(u[3])
  Fcn1 : Fcn  Expr=-u[1]*sin(u[3]) + u[2]*cos(u[3])
  Mux : Mux  Inputs=3
  Mux1 : Mux  Inputs=[2 1]
  Mux2 : Mux  Inputs=[2 1]
  Selector : Selector  InputPortWidth=3  IndexOptions=Index vector (dialog)  Indices=[1 2]  OutputSizes=1
  Selector1 : Selector  InputPortWidth=3  IndexOptions=Index vector (dialog)  Indices=[3]  OutputSizes=1
  dq : Outport  InitialOutput=[0,0]  VectorParamsAs1DForOutWhenUnconnected=off
  wires:
  alpha_beta/1 -> Selector/1, Selector1/1
  Mux1/1 -> Fcn/1
  Fcn1/1 -> Mux/2
  Fcn/1 -> Mux/1
  wtNow/1 -> Mux2/2, Mux1/2
  Mux/1 -> dq/1
  Mux2/1 -> Fcn1/1
  Selector/1 -> Mux2/1, Mux1/1
  Selector1/1 -> Mux/3

== system GCI_Ctrl_PLL_C2000/C2000_SW/CtrlLoop/PLL_Vref/Subsystem/dd_dqz1/Subsystem2 ==
  note: [  al
      |     be  ]
  note: q = -al*sin(wt) + be*cos(wt)
  note: [  cos(wt)   sin(wt)
      |    -sin(wt)    cos(wt)   ]
  note: d = al*cos(wt) + be*sin(wt)
  note: [ d
      |    q ]
  note: *
  note: =
  alpha_beta : Inport
  wtNow : Inport  Port=2  PortDimensions=1
  Fcn : Fcn  Expr=u[1]*cos(u[3]) + u[2]*sin(u[3])
  Fcn1 : Fcn  Expr=-u[1]*sin(u[3]) + u[2]*cos(u[3])
  Mux : Mux  Inputs=3
  Mux1 : Mux  Inputs=[2 1]
  Mux2 : Mux  Inputs=[2 1]
  Selector : Selector  InputPortWidth=3  IndexOptions=Index vector (dialog)  Indices=[1 2]  OutputSizes=1
  Selector1 : Selector  InputPortWidth=3  IndexOptions=Index vector (dialog)  Indices=[3]  OutputSizes=1
  dq : Outport  InitialOutput=[0,0]  VectorParamsAs1DForOutWhenUnconnected=off
  wires:
  Selector1/1 -> Mux/3
  Selector/1 -> Mux1/1, Mux2/1
  Mux2/1 -> Fcn1/1
  Mux/1 -> dq/1
  Fcn/1 -> Mux/1
  Fcn1/1 -> Mux/2
  Mux1/1 -> Fcn/1
  alpha_beta/1 -> Selector1/1, Selector/1
  wtNow/1 -> Mux2/2, Mux1/2

== system GCI_Ctrl_PLL_C2000/C2000_SW/CtrlLoop/PLL_Vref/Subsystem/dd_dqz1/Subsystem3 ==
  Vdq_in : Inport
  Vdq_Inverse : Inport  Port=2
  Theta : Inport  Port=3
  Cos : Trigonometry  Operator=cos
  Demux1 : Demux  Outputs=2
  Demux2 : Demux  Outputs=2
  Gain : Gain  Gain=2  ParamDataTypeStr=single
  Ground : Ground
  Mux : Mux  Inputs=3
  Product{,1..3} (4 alike) : Product
  Selector : Selector  InputPortWidth=3  IndexOptions=Index vector (dialog)  Indices=[1 2]  OutputSizes=1
  Selector1 : Selector  InputPortWidth=3  IndexOptions=Index vector (dialog)  Indices=[1 2]  OutputSizes=1
  Sin : Trigonometry
  Sum : Sum  Inputs=|+-
  Sum1 : Sum  Inputs=|++
  Sum2 : Sum  Inputs=|+-
  Sum3 : Sum  Inputs=|+-
  Vdq_out : Outport  VectorParamsAs1DForOutWhenUnconnected=off
  wires:
  Ground/1 -> Mux/3
  Mux/1 -> Vdq_out/1
  Sum3/1 -> Mux/2
  Product3/1 -> Sum3/2
  Sum1/1 -> Sum3/1
  [Vq_Neg] -> Product3/1
  [Cos] -> Product3/2
  Product2/1 -> Sum2/2
  [Vq_Neg] -> Product2/1
  [Sin] -> Product2/2
  Sum2/1 -> Mux/1
  Sum/1 -> Sum2/1
  [Vq_Pos] -> Sum1/1
  Product1/1 -> Sum1/2
  [Vd_Neg] -> Product1/1
  [Sin] -> Product1/2
  [Cos] -> Product/2
  [Vd_Neg] -> Product/1
  Product/1 -> Sum/2
  Cos/1 -> [Cos]
  Sin/1 -> [Sin]
  [Vd_Pos] -> Sum/1
  Demux1/2 -> [Vq_Neg]
  Demux1/1 -> [Vd_Neg]
  Demux2/2 -> [Vq_Pos]
  Demux2/1 -> [Vd_Pos]
  Vdq_Inverse/1 -> Selector1/1
  Selector1/1 -> Demux1/1
  Selector/1 -> Demux2/1
  Vdq_in/1 -> Selector/1
  Gain/1 -> Sin/1, Cos/1
  Theta/1 -> Gain/1

== system GCI_Ctrl_PLL_C2000/C2000_SW/CtrlLoop/PLL_Vref/Subsystem/dd_dqz1/Subsystem4 ==
  Vdq_in : Inport
  Vdq_Inverse : Inport  Port=2
  Theta : Inport  Port=3
  Cos : Trigonometry  Operator=cos
  Demux1 : Demux  Outputs=2
  Demux2 : Demux  Outputs=2
  Gain : Gain  Gain=2  ParamDataTypeStr=single
  Ground : Ground
  Mux : Mux  Inputs=3
  Product{,1..3} (4 alike) : Product
  Selector : Selector  InputPortWidth=3  IndexOptions=Index vector (dialog)  Indices=[1 2]  OutputSizes=1
  Selector1 : Selector  InputPortWidth=3  IndexOptions=Index vector (dialog)  Indices=[1 2]  OutputSizes=1
  Sin : Trigonometry
  Sum : Sum  Inputs=|+-
  Sum1 : Sum  Inputs=|++
  Sum2 : Sum  Inputs=|+-
  Sum3 : Sum  Inputs=|+-
  Vdq_out : Outport  VectorParamsAs1DForOutWhenUnconnected=off
  wires:
  Theta/1 -> Gain/1
  Gain/1 -> Cos/1, Sin/1
  Vdq_in/1 -> Selector/1
  Selector/1 -> Demux2/1
  Selector1/1 -> Demux1/1
  Vdq_Inverse/1 -> Selector1/1
  Demux2/1 -> [Vd_Pos]
  Demux2/2 -> [Vq_Pos]
  Demux1/1 -> [Vd_Neg]
  Demux1/2 -> [Vq_Neg]
  [Vd_Pos] -> Sum/1
  Sin/1 -> [Sin]
  Cos/1 -> [Cos]
  Product/1 -> Sum/2
  [Vd_Neg] -> Product/1
  [Cos] -> Product/2
  [Sin] -> Product1/2
  [Vd_Neg] -> Product1/1
  Product1/1 -> Sum1/2
  [Vq_Pos] -> Sum1/1
  Sum/1 -> Sum2/1
  Sum2/1 -> Mux/1
  [Sin] -> Product2/2
  [Vq_Neg] -> Product2/1
  Product2/1 -> Sum2/2
  [Cos] -> Product3/2
  [Vq_Neg] -> Product3/1
  Sum1/1 -> Sum3/1
  Product3/1 -> Sum3/2
  Sum3/1 -> Mux/2
  Mux/1 -> Vdq_out/1
  Ground/1 -> Mux/3

== system GCI_Ctrl_PLL_C2000/C2000_SW/CtrlLoop/PLL_Vref/Subsystem/dd_dqz2/LPF ==
  u : Inport
  Alpha : Gain  Gain=(2-w*Ts)/(2+w*Ts)
  Beta : Gain  Gain=(w*Ts)/(2+w*Ts)
  Delay1 : Delay  DelayLength=1  InitialCondition=y_0
  Delay2 : Delay  DelayLength=1
  Sum1 : Sum  Inputs=++|
  Sum2 : Sum  Inputs=|++
  y : Outport  VectorParamsAs1DForOutWhenUnconnected=off
  wires:
  u/1 -> Sum1/1, Delay2/1
  Delay1/1 -> Alpha/1  "y(n-1)"
  Alpha/1 -> Sum2/2
  Delay2/1 -> Sum1/2
  Sum1/1 -> Beta/1
  Beta/1 -> Sum2/1
  Sum2/1 -> Delay1/1, y/1

== system GCI_Ctrl_PLL_C2000/C2000_SW/CtrlLoop/PLL_Vref/Subsystem/dd_dqz2/LPF1 ==
  u : Inport
  Alpha : Gain  Gain=(2-w*Ts)/(2+w*Ts)
  Beta : Gain  Gain=(w*Ts)/(2+w*Ts)
  Delay1 : Delay  DelayLength=1  InitialCondition=y_0
  Delay2 : Delay  DelayLength=1
  Sum1 : Sum  Inputs=++|
  Sum2 : Sum  Inputs=|++
  y : Outport  VectorParamsAs1DForOutWhenUnconnected=off
  wires:
  Sum2/1 -> y/1, Delay1/1
  Beta/1 -> Sum2/1
  Sum1/1 -> Beta/1
  Delay2/1 -> Sum1/2
  Alpha/1 -> Sum2/2
  Delay1/1 -> Alpha/1  "y(n-1)"
  u/1 -> Delay2/1, Sum1/1

== system GCI_Ctrl_PLL_C2000/C2000_SW/CtrlLoop/PLL_Vref/Subsystem/dd_dqz2/Subsystem ==
  abc : Inport  PortDimensions=3
  Gain1 : Gain  Gain=single(2/3)  ParamDataTypeStr=single  SaturateOnIntegerOverflow=on  OutDataTypeStr=Inherit: Same as input
  Gain3 : Gain  Gain="single([ 1   -1/2   -1/2; 0   sqrt(3)/2   -sqrt(3)/2; 1/2  1/2  1/2 ] )"  Multiplication=Matrix(K*u) (u vector)  ParamDataTypeStr=single  SaturateOnIntegerOverflow=on  OutDataTypeStr=Inherit: Same as input
  al_be_0 : Outport  VectorParamsAs1DForOutWhenUnconnected=off
  wires:
  Gain1/1 -> al_be_0/1  "AlphaBetaZero"
  Gain3/1 -> Gain1/1
  abc/1 -> Gain3/1

== system GCI_Ctrl_PLL_C2000/C2000_SW/CtrlLoop/PLL_Vref/Subsystem/dd_dqz2/Subsystem1 ==
  note: [  al
      |     be  ]
  note: q = -al*sin(wt) + be*cos(wt)
  note: [  cos(wt)   sin(wt)
      |    -sin(wt)    cos(wt)   ]
  note: d = al*cos(wt) + be*sin(wt)
  note: [ d
      |    q ]
  note: *
  note: =
  alpha_beta : Inport
  wtNow : Inport  Port=2  PortDimensions=1
  Fcn : Fcn  Expr=u[1]*cos(u[3]) + u[2]*sin(u[3])
  Fcn1 : Fcn  Expr=-u[1]*sin(u[3]) + u[2]*cos(u[3])
  Mux : Mux  Inputs=3
  Mux1 : Mux  Inputs=[2 1]
  Mux2 : Mux  Inputs=[2 1]
  Selector : Selector  InputPortWidth=3  IndexOptions=Index vector (dialog)  Indices=[1 2]  OutputSizes=1
  Selector1 : Selector  InputPortWidth=3  IndexOptions=Index vector (dialog)  Indices=[3]  OutputSizes=1
  dq : Outport  InitialOutput=[0,0]  VectorParamsAs1DForOutWhenUnconnected=off
  wires:
  Selector1/1 -> Mux/3
  Selector/1 -> Mux1/1, Mux2/1
  Mux2/1 -> Fcn1/1
  Mux/1 -> dq/1  "dq"
  wtNow/1 -> Mux1/2, Mux2/2
  Fcn/1 -> Mux/1
  Fcn1/1 -> Mux/2
  Mux1/1 -> Fcn/1
  alpha_beta/1 -> Selector1/1, Selector/1

== system GCI_Ctrl_PLL_C2000/C2000_SW/CtrlLoop/PLL_Vref/Subsystem/dd_dqz2/Subsystem2 ==
  note: =
  note: *
  note: [ d
      |    q ]
  note: d = al*cos(wt) + be*sin(wt)
  note: [  cos(wt)   sin(wt)
      |    -sin(wt)    cos(wt)   ]
  note: q = -al*sin(wt) + be*cos(wt)
  note: [  al
      |     be  ]
  alpha_beta : Inport
  wtNow : Inport  Port=2  PortDimensions=1
  Fcn : Fcn  Expr=u[1]*cos(u[3]) + u[2]*sin(u[3])
  Fcn1 : Fcn  Expr=-u[1]*sin(u[3]) + u[2]*cos(u[3])
  Mux : Mux  Inputs=3
  Mux1 : Mux  Inputs=[2 1]
  Mux2 : Mux  Inputs=[2 1]
  Selector : Selector  InputPortWidth=3  IndexOptions=Index vector (dialog)  Indices=[1 2]  OutputSizes=1
  Selector1 : Selector  InputPortWidth=3  IndexOptions=Index vector (dialog)  Indices=[3]  OutputSizes=1
  dq : Outport  InitialOutput=[0,0]  VectorParamsAs1DForOutWhenUnconnected=off
  wires:
  alpha_beta/1 -> Selector/1, Selector1/1
  Mux1/1 -> Fcn/1
  Fcn1/1 -> Mux/2
  Fcn/1 -> Mux/1
  wtNow/1 -> Mux2/2, Mux1/2
  Mux/1 -> dq/1  "dq"
  Mux2/1 -> Fcn1/1
  Selector/1 -> Mux2/1, Mux1/1
  Selector1/1 -> Mux/3

== system GCI_Ctrl_PLL_C2000/C2000_SW/CtrlLoop/PLL_Vref/Subsystem/dd_dqz2/Subsystem3 ==
  Vdq_in : Inport
  Vdq_Inverse : Inport  Port=2
  Theta : Inport  Port=3
  Cos : Trigonometry  Operator=cos
  Demux1 : Demux  Outputs=2
  Demux2 : Demux  Outputs=2
  Gain : Gain  Gain=2  ParamDataTypeStr=single
  Ground : Ground
  Mux : Mux  Inputs=3
  Product{,1..3} (4 alike) : Product
  Selector : Selector  InputPortWidth=3  IndexOptions=Index vector (dialog)  Indices=[1 2]  OutputSizes=1
  Selector1 : Selector  InputPortWidth=3  IndexOptions=Index vector (dialog)  Indices=[1 2]  OutputSizes=1
  Sin : Trigonometry
  Sum : Sum  Inputs=|+-
  Sum1 : Sum  Inputs=|++
  Sum2 : Sum  Inputs=|+-
  Sum3 : Sum  Inputs=|+-
  Vdq_out : Outport  VectorParamsAs1DForOutWhenUnconnected=off
  wires:
  Theta/1 -> Gain/1
  Gain/1 -> Cos/1, Sin/1
  Vdq_in/1 -> Selector/1
  Selector/1 -> Demux2/1
  Selector1/1 -> Demux1/1
  Vdq_Inverse/1 -> Selector1/1
  Demux2/1 -> [Vd_Pos]
  Demux2/2 -> [Vq_Pos]
  Demux1/1 -> [Vd_Neg]
  Demux1/2 -> [Vq_Neg]
  [Vd_Pos] -> Sum/1
  Sin/1 -> [Sin]
  Cos/1 -> [Cos]
  Product/1 -> Sum/2
  [Vd_Neg] -> Product/1
  [Cos] -> Product/2
  [Sin] -> Product1/2
  [Vd_Neg] -> Product1/1
  Product1/1 -> Sum1/2
  [Vq_Pos] -> Sum1/1
  Sum/1 -> Sum2/1
  Sum2/1 -> Mux/1
  [Sin] -> Product2/2
  [Vq_Neg] -> Product2/1
  Product2/1 -> Sum2/2
  [Cos] -> Product3/2
  [Vq_Neg] -> Product3/1
  Sum1/1 -> Sum3/1
  Product3/1 -> Sum3/2
  Sum3/1 -> Mux/2
  Mux/1 -> Vdq_out/1
  Ground/1 -> Mux/3

== system GCI_Ctrl_PLL_C2000/C2000_SW/CtrlLoop/PLL_Vref/Subsystem/dd_dqz2/Subsystem4 ==
  Vdq_in : Inport
  Vdq_Inverse : Inport  Port=2
  Theta : Inport  Port=3
  Cos : Trigonometry  Operator=cos
  Demux1 : Demux  Outputs=2
  Demux2 : Demux  Outputs=2
  Gain : Gain  Gain=2  ParamDataTypeStr=single
  Ground : Ground
  Mux : Mux  Inputs=3
  Product{,1..3} (4 alike) : Product
  Selector : Selector  InputPortWidth=3  IndexOptions=Index vector (dialog)  Indices=[1 2]  OutputSizes=1
  Selector1 : Selector  InputPortWidth=3  IndexOptions=Index vector (dialog)  Indices=[1 2]  OutputSizes=1
  Sin : Trigonometry
  Sum : Sum  Inputs=|+-
  Sum1 : Sum  Inputs=|++
  Sum2 : Sum  Inputs=|+-
  Sum3 : Sum  Inputs=|+-
  Vdq_out : Outport  VectorParamsAs1DForOutWhenUnconnected=off
  wires:
  Ground/1 -> Mux/3
  Mux/1 -> Vdq_out/1
  Sum3/1 -> Mux/2
  Product3/1 -> Sum3/2
  Sum1/1 -> Sum3/1
  [Vq_Neg] -> Product3/1
  [Cos] -> Product3/2
  Product2/1 -> Sum2/2
  [Vq_Neg] -> Product2/1
  [Sin] -> Product2/2
  Sum2/1 -> Mux/1
  Sum/1 -> Sum2/1
  [Vq_Pos] -> Sum1/1
  Product1/1 -> Sum1/2
  [Vd_Neg] -> Product1/1
  [Sin] -> Product1/2
  [Cos] -> Product/2
  [Vd_Neg] -> Product/1
  Product/1 -> Sum/2
  Cos/1 -> [Cos]
  Sin/1 -> [Sin]
  [Vd_Pos] -> Sum/1
  Demux1/2 -> [Vq_Neg]
  Demux1/1 -> [Vd_Neg]
  Demux2/2 -> [Vq_Pos]
  Demux2/1 -> [Vd_Pos]
  Vdq_Inverse/1 -> Selector1/1
  Selector1/1 -> Demux1/1
  Selector/1 -> Demux2/1
  Vdq_in/1 -> Selector/1
  Gain/1 -> Sin/1, Cos/1
  Theta/1 -> Gain/1

== system GCI_Ctrl_PLL_C2000/C2000_SW/CtrlLoop/PLL_Vref/abc2dqzFilt/Single_SOGI/Subsystem1 ==
  AlphBeta : Inport
  w : Inport  Port=2
  Gain : Gain  Gain=single(1)  ParamDataTypeStr=single
  Gain1 : Gain  Gain=single(1)  ParamDataTypeStr=single
  Ground : Ground
  Mux : Mux  Inputs=3
  SOGI_QSG : Subsystem
  Selector1 : Selector  InputPortWidth=3  IndexOptions=Index vector (dialog)  Indices=[1]  OutputSizes=1
  AlphBetaCor : Outport  VectorParamsAs1DForOutWhenUnconnected=off
  wires:
  Gain1/1 -> Mux/2
  Gain/1 -> Mux/1
  w/1 -> SOGI_QSG/2(wo)
  Mux/1 -> AlphBetaCor/1
  Ground/1 -> Mux/3
  SOGI_QSG/2(qY) -> Gain1/1
  Selector1/1 -> SOGI_QSG/1(U)
  AlphBeta/1 -> Selector1/1
  SOGI_QSG/1(Y) -> Gain/1

== system GCI_Ctrl_PLL_C2000/C2000_SW/CtrlLoop/PLL_Vref/abc2dqzFilt/Single_SOGI/Subsystem2 ==
  note: [  al
      |     be  ]
  note: q = -al*sin(wt) + be*cos(wt)
  note: [  cos(wt)   sin(wt)
      |    -sin(wt)    cos(wt)   ]
  note: d = al*cos(wt) + be*sin(wt)
  note: [ d
      |    q ]
  note: *
  note: =
  alpha_beta : Inport
  Ang : Inport  Port=2  PortDimensions=1
  Fcn : Fcn  Expr=u[1]*cos(u[3]) + u[2]*sin(u[3])
  Fcn1 : Fcn  Expr=-u[1]*sin(u[3]) + u[2]*cos(u[3])
  Mux : Mux  Inputs=3
  Mux1 : Mux  Inputs=[2 1]
  Mux2 : Mux  Inputs=[2 1]
  Selector : Selector  InputPortWidth=3  IndexOptions=Index vector (dialog)  Indices=[1 2]  OutputSizes=1
  Selector1 : Selector  InputPortWidth=3  IndexOptions=Index vector (dialog)  Indices=[3]  OutputSizes=1
  dq : Outport  InitialOutput=[0,0]  VectorParamsAs1DForOutWhenUnconnected=off
  wires:
  Selector1/1 -> Mux/3
  Selector/1 -> Mux1/1, Mux2/1
  Mux2/1 -> Fcn1/1
  Mux/1 -> dq/1
  Ang/1 -> Mux1/2, Mux2/2
  Fcn/1 -> Mux/1
  Fcn1/1 -> Mux/2
  Mux1/1 -> Fcn/1
  alpha_beta/1 -> Selector1/1, Selector/1

== system GCI_Ctrl_PLL_C2000/C2000_SW/CtrlLoop/PLL_Vref/abc2dqzFilt/Single_SOGI/Subsystem3 ==
  note: =
  note: *
  note: [ d
      |    q ]
  note: d = al*cos(wt) + be*sin(wt)
  note: [  cos(wt)   sin(wt)
      |    -sin(wt)    cos(wt)   ]
  note: q = -al*sin(wt) + be*cos(wt)
  note: [  al
      |     be  ]
  alpha_beta : Inport
  Ang : Inport  Port=2  PortDimensions=1
  Fcn : Fcn  Expr=u[1]*cos(u[3]) + u[2]*sin(u[3])
  Fcn1 : Fcn  Expr=-u[1]*sin(u[3]) + u[2]*cos(u[3])
  Mux : Mux  Inputs=3
  Mux1 : Mux  Inputs=[2 1]
  Mux2 : Mux  Inputs=[2 1]
  Selector : Selector  InputPortWidth=3  IndexOptions=Index vector (dialog)  Indices=[1 2]  OutputSizes=1
  Selector1 : Selector  InputPortWidth=3  IndexOptions=Index vector (dialog)  Indices=[3]  OutputSizes=1
  dq : Outport  InitialOutput=[0,0]  VectorParamsAs1DForOutWhenUnconnected=off
  wires:
  alpha_beta/1 -> Selector/1, Selector1/1
  Mux1/1 -> Fcn/1
  Fcn1/1 -> Mux/2
  Fcn/1 -> Mux/1
  Ang/1 -> Mux2/2, Mux1/2
  Mux/1 -> dq/1
  Mux2/1 -> Fcn1/1
  Selector/1 -> Mux2/1, Mux1/1
  Selector1/1 -> Mux/3

== system GCI_Ctrl_PLL_C2000/C2000_SW/CtrlLoop/PLL_Vref/abc2dqzFilt/dd_dqz/LPF1 ==
  u : Inport
  Alpha : Gain  Gain=(2-w*Ts)/(2+w*Ts)
  Beta : Gain  Gain=(w*Ts)/(2+w*Ts)
  Delay1 : Delay  DelayLength=1  InitialCondition=y_0
  Delay2 : Delay  DelayLength=1
  Sum1 : Sum  Inputs=++|
  Sum2 : Sum  Inputs=|++
  y : Outport  VectorParamsAs1DForOutWhenUnconnected=off
  wires:
  Sum2/1 -> y/1, Delay1/1
  Beta/1 -> Sum2/1
  Sum1/1 -> Beta/1
  Delay2/1 -> Sum1/2
  Alpha/1 -> Sum2/2
  Delay1/1 -> Alpha/1  "y(n-1)"
  u/1 -> Delay2/1, Sum1/1

== system GCI_Ctrl_PLL_C2000/C2000_SW/CtrlLoop/PLL_Vref/abc2dqzFilt/dd_dqz/LPF2 ==
  u : Inport
  Alpha : Gain  Gain=(2-w*Ts)/(2+w*Ts)
  Beta : Gain  Gain=(w*Ts)/(2+w*Ts)
  Delay1 : Delay  DelayLength=1  InitialCondition=y_0
  Delay2 : Delay  DelayLength=1
  Sum1 : Sum  Inputs=++|
  Sum2 : Sum  Inputs=|++
  y : Outport  VectorParamsAs1DForOutWhenUnconnected=off
  wires:
  u/1 -> Sum1/1, Delay2/1
  Delay1/1 -> Alpha/1  "y(n-1)"
  Alpha/1 -> Sum2/2
  Delay2/1 -> Sum1/2
  Sum1/1 -> Beta/1
  Beta/1 -> Sum2/1
  Sum2/1 -> Delay1/1, y/1

== system GCI_Ctrl_PLL_C2000/C2000_SW/CtrlLoop/PLL_Vref/abc2dqzFilt/dd_dqz/Subsystem ==
  abc : Inport  PortDimensions=3
  Gain1 : Gain  Gain=single(2/3)  ParamDataTypeStr=single  SaturateOnIntegerOverflow=on  OutDataTypeStr=Inherit: Same as input
  Gain3 : Gain  Gain="single([ 1   -1/2   -1/2; 0   sqrt(3)/2   -sqrt(3)/2; 1/2  1/2  1/2 ] )"  Multiplication=Matrix(K*u) (u vector)  ParamDataTypeStr=single  SaturateOnIntegerOverflow=on  OutDataTypeStr=Inherit: Same as input
  al_be_0 : Outport  VectorParamsAs1DForOutWhenUnconnected=off
  wires:
  Gain1/1 -> al_be_0/1
  Gain3/1 -> Gain1/1
  abc/1 -> Gain3/1

== system GCI_Ctrl_PLL_C2000/C2000_SW/CtrlLoop/PLL_Vref/abc2dqzFilt/dd_dqz/Subsystem1 ==
  note: [  al
      |     be  ]
  note: q = -al*sin(wt) + be*cos(wt)
  note: [  cos(wt)   sin(wt)
      |    -sin(wt)    cos(wt)   ]
  note: d = al*cos(wt) + be*sin(wt)
  note: [ d
      |    q ]
  note: *
  note: =
  alpha_beta : Inport
  Ang : Inport  Port=2  PortDimensions=1
  Fcn : Fcn  Expr=u[1]*cos(u[3]) + u[2]*sin(u[3])
  Fcn1 : Fcn  Expr=-u[1]*sin(u[3]) + u[2]*cos(u[3])
  Mux : Mux  Inputs=3
  Mux1 : Mux  Inputs=[2 1]
  Mux2 : Mux  Inputs=[2 1]
  Selector : Selector  InputPortWidth=3  IndexOptions=Index vector (dialog)  Indices=[1 2]  OutputSizes=1
  Selector1 : Selector  InputPortWidth=3  IndexOptions=Index vector (dialog)  Indices=[3]  OutputSizes=1
  dq : Outport  InitialOutput=[0,0]  VectorParamsAs1DForOutWhenUnconnected=off
  wires:
  Selector1/1 -> Mux/3
  Selector/1 -> Mux1/1, Mux2/1
  Mux2/1 -> Fcn1/1
  Mux/1 -> dq/1
  Ang/1 -> Mux1/2, Mux2/2
  Fcn/1 -> Mux/1
  Fcn1/1 -> Mux/2
  Mux1/1 -> Fcn/1
  alpha_beta/1 -> Selector1/1, Selector/1

== system GCI_Ctrl_PLL_C2000/C2000_SW/CtrlLoop/PLL_Vref/abc2dqzFilt/dd_dqz/Subsystem2 ==
  note: =
  note: *
  note: [ d
      |    q ]
  note: d = al*cos(wt) + be*sin(wt)
  note: [  cos(wt)   sin(wt)
      |    -sin(wt)    cos(wt)   ]
  note: q = -al*sin(wt) + be*cos(wt)
  note: [  al
      |     be  ]
  alpha_beta : Inport
  Ang : Inport  Port=2  PortDimensions=1
  Fcn : Fcn  Expr=u[1]*cos(u[3]) + u[2]*sin(u[3])
  Fcn1 : Fcn  Expr=-u[1]*sin(u[3]) + u[2]*cos(u[3])
  Mux : Mux  Inputs=3
  Mux1 : Mux  Inputs=[2 1]
  Mux2 : Mux  Inputs=[2 1]
  Selector : Selector  InputPortWidth=3  IndexOptions=Index vector (dialog)  Indices=[1 2]  OutputSizes=1
  Selector1 : Selector  InputPortWidth=3  IndexOptions=Index vector (dialog)  Indices=[3]  OutputSizes=1
  dq : Outport  InitialOutput=[0,0]  VectorParamsAs1DForOutWhenUnconnected=off
  wires:
  alpha_beta/1 -> Selector/1, Selector1/1
  Mux1/1 -> Fcn/1
  Fcn1/1 -> Mux/2
  Fcn/1 -> Mux/1
  Ang/1 -> Mux2/2, Mux1/2
  Mux/1 -> dq/1
  Mux2/1 -> Fcn1/1
  Selector/1 -> Mux2/1, Mux1/1
  Selector1/1 -> Mux/3
